simulink model "math_complex_test"  (Simulink 8.4)
settings: Solver=VariableStepDiscrete  StartTime=0.0  StopTime=10.0  RelTol=1e-3
undefined symbols (not defined in the file or in its folder): magnitude
settings Model: Creator=arnaud  LastModifiedBy=arnaud
settings DataIOCC: SaveFormat=Structure

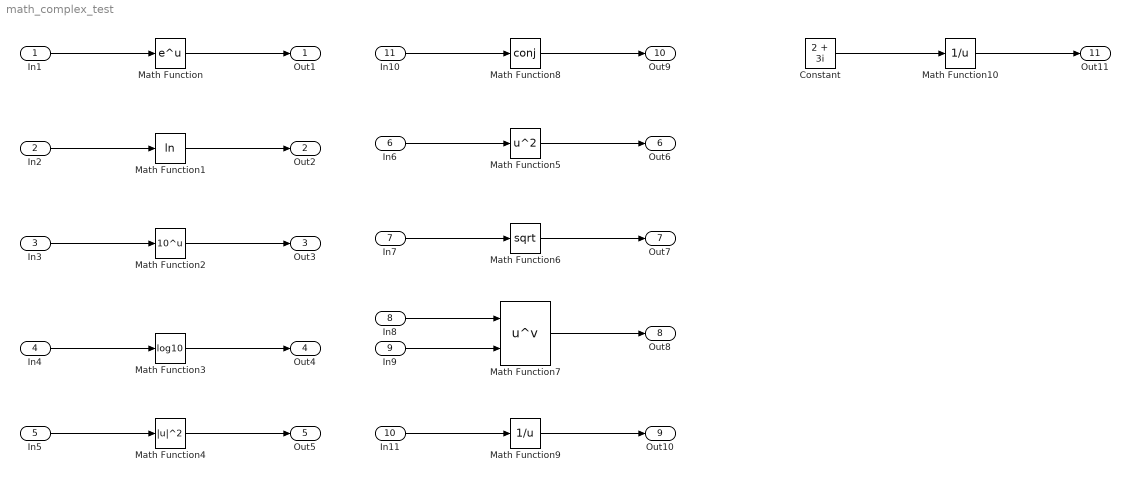
== system math_complex_test ==
  In1 : Inport
      settings: SignalType=complex
  In2 : Inport  Port=2
      settings: SignalType=complex
  In3 : Inport  Port=3
      settings: SignalType=complex
  In4 : Inport  Port=4
      settings: SignalType=complex
  In5 : Inport  Port=5
      settings: SignalType=complex
  In6 : Inport  Port=6
      settings: SignalType=complex
  In7 : Inport  Port=7
      settings: SignalType=complex
  In8 : Inport  Port=8
      settings: SignalType=complex
  In9 : Inport  Port=9
      settings: SignalType=complex
  In11 : Inport  Port=10
      settings: SignalType=complex
  In10 : Inport  Port=11
      settings: SignalType=complex
  Constant : Constant  Value=2 + 3i
  Math Function : Math  SaturateOnIntegerOverflow=on
  Math Function1 : Math  Operator=log  SaturateOnIntegerOverflow=on
  Math Function10 : Math  Operator=reciprocal  SaturateOnIntegerOverflow=on
  Math Function2 : Math  Operator=10^u  SaturateOnIntegerOverflow=on
  Math Function3 : Math  Operator=log10  SaturateOnIntegerOverflow=on
  Math Function4 : Math  Operator=magnitude^2  SaturateOnIntegerOverflow=on
  Math Function5 : Math  Operator=square  SaturateOnIntegerOverflow=on
  Math Function6 : Math  Operator=sqrt  SaturateOnIntegerOverflow=on
  Math Function7 : Math  Operator=pow  SaturateOnIntegerOverflow=on
  Math Function8 : Math  Operator=conj  SaturateOnIntegerOverflow=on
  Math Function9 : Math  Operator=reciprocal  SaturateOnIntegerOverflow=on
  Out1 : Outport
  Out2 : Outport  Port=2
  Out3 : Outport  Port=3
  Out4 : Outport  Port=4
  Out5 : Outport  Port=5
  Out6 : Outport  Port=6
  Out7 : Outport  Port=7
  Out8 : Outport  Port=8
  Out10 : Outport  Port=9
  Out9 : Outport  Port=10
  Out11 : Outport  Port=11
  wires:
  In1/1 -> Math Function/1
  Math Function/1 -> Out1/1
  In2/1 -> Math Function1/1
  Math Function1/1 -> Out2/1
  In3/1 -> Math Function2/1
  Math Function2/1 -> Out3/1
  In4/1 -> Math Function3/1
  Math Function3/1 -> Out4/1
  In5/1 -> Math Function4/1
  Math Function4/1 -> Out5/1
  In6/1 -> Math Function5/1
  Math Function5/1 -> Out6/1
  In7/1 -> Math Function6/1
  Math Function6/1 -> Out7/1
  In8/1 -> Math Function7/1
  In9/1 -> Math Function7/2
  Math Function7/1 -> Out8/1
  In11/1 -> Math Function9/1
  Math Function9/1 -> Out10/1
  In10/1 -> Math Function8/1
  Math Function8/1 -> Out9/1
  Constant/1 -> Math Function10/1
  Math Function10/1 -> Out11/1
